simulink model "SPHERE_model4_Fuzzy"  (R2020a)
settings: Solver=ode4  StartTime=0.0  StopTime=30  FixedStep=0.01428571  RelTol=1e-3
values from neighbouring files (symbols this model uses):
  Final_val = 18    [Initial_script.m]    (also in Initial_script_test.m = -28; Initial_script_test2.m = -28)
  K = 25.937    [Initial_script.m]    (also in Initial_script_test.m; Initial_script_test2.m)
  L = -[ M2*l*(-2*l + R) - 2*J2, 0, -2*M2*l*g ]    [Initial_script.m]    (also in Initial_script_test.m; Initial_script_test2.m)
  M = [ J1 + 2*J2 + M1*R^2 + M2*(2*l^2 - 3*R*l + R^2), -Tv, 2*l*g*M2 ]    [Initial_script.m]    (also in Initial_script_test.m; Initial_script_test2.m)
  Smax = 502    [Initial_script.m]    (also in Initial_script_test.m; Initial_script_test2.m)
  Smin = -480    [Initial_script.m]    (also in Initial_script_test.m; Initial_script_test2.m)
  Step_time = 3.18    [Initial_script.m]    (also in Initial_script_test.m = 4.45; Initial_script_test2.m = 4.5)
  Top = 0.015    [Initial_script.m]    (also in Initial_script_test.m; Initial_script_test2.m)
undefined symbols (not defined in the file or in its folder): sigbuilder_block
libraries: fuzblock x1
settings Model: Creator=Adrian  LastModifiedBy=Adrian
settings OptimizationCC: DefaultParameterBehavior=Inlined  EnhancedBackFolding=on  PassReuseOutputArgsAs=Individual arguments  ZeroExternalMemoryAtStartup=off  ZeroInternalMemoryAtStartup=off  OptimizeBlockOrder=speed  DifferentSizesBufferReuse=on  OptimizationCustomize=off  EfficientTunableParamExpr=on
settings DebuggingCC: ParameterTunabilityLossMsg=error
settings SFSimCC: MATLABDynamicMemAlloc=off
settings RTWCC: SystemTargetFile=ert.tlc  TemplateMakefile=ert_default_tmf
settings CodeAppCC: ForceParamTrailComments=on  IgnoreCustomStorageClasses=off  OperatorAnnotations=on  SimulinkDataObjDesc=on  SFDataObjDesc=on  InsertBlockDesc=on
settings ERTTargetCC: TargetLangStandard=C99 (ISO)  GenerateSampleERTMain=on  InlinedParameterPlacement=NonHierarchical  ERTCustomFileTemplate=example_file_process.tlc

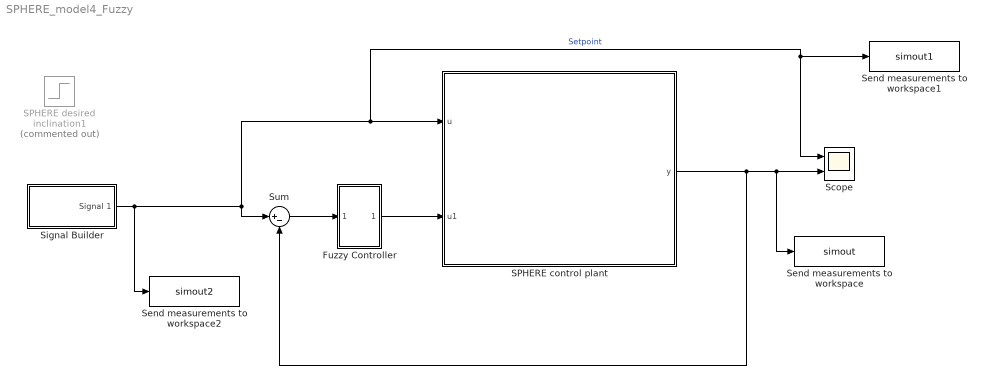
== system SPHERE_model4_Fuzzy ==
  Fuzzy Controller : Subsystem
  SPHERE control plant : Subsystem
      mask Display: image('C:\Users\Adrian\Documents\Praca Magisterska\Robot kulisty by Adrian\Praca Magisterska\LaTex\Pictures\Old\sphere_full.PNG'); % Use "Edit Image" on toolstrip to change.
  SPHERE desired inclination1 : Step  Commented=on  Time=Step_time  After=Final_val  SampleTime=0
  Scope : Scope  NumInputPorts=2
  Send measurements to workspace : ToWorkspace  VariableName=simout  SaveFormat=Timeseries  SampleTime=-1
  Send measurements to workspace1 : ToWorkspace  VariableName=simout1  SaveFormat=Timeseries  SampleTime=-1
  Send measurements to workspace2 : ToWorkspace  VariableName=simout2  SaveFormat=Timeseries  SampleTime=-1
  Signal Builder : Subsystem  Tag=STV Subsys  LoadFcn=sigbuilder_block('load');  StartFcn=sigbuilder_block('start');  StopFcn=sigbuilder_block('stop');  ClipboardFcn=sigbuilder_block('clipboard');  mask(Sigbuilder block){tuvar=[0:10]}
      mask help: Simulink:masks:SigbuilderBlock_MD
      mask init:
      | if ~strcmp(get_param(bdroot(gcbh),'SimulationStatus'),'stopped') tuvar = sigbuilder_block('maskInit'); end
      settings: CopyFcn=sigbuilder_block('copy');  DeleteFcn=sigbuilder_block('delete');  ModelCloseFcn=sigbuilder_block('modelClose');  PreSaveFcn=sigbuilder_block('preSave');  PauseFcn=sigbuilder_block('pause');  ContinueFcn=sigbuilder_block('continue');  NameChangeFcn=sigbuilder_block('namechange');  OpenFcn=sigbuilder_block('open',[90.75 122.25 550.5 399.75 ]);  CloseFcn=sigbuilder_block('close');
      mask Display: plot(0, 0, 100, 100,[2, 2, 32, 32, 2], [68, 8, 8, 68, 68],[32, 2], [38, 38], [32, 19, 2],[53, 60, 44], [32, 17, 17, 2],[16, 16, 31, 31]);txt = getActiveGroup(gcbh);text(2, 100, txt,'verticalAlignment', 'top');
  Sum : Sum  Inputs=|+-
  wires:
  SPHERE control plant/1(y) -> Sum/2, Send measurements to workspace/1, Scope/2
  Signal Builder/1(Signal 1) -> Send measurements to workspace2/1, Sum/1, Send measurements to workspace1/1, Scope/1, SPHERE control plant/1(u)  "Setpoint"
  Sum/1 -> Fuzzy Controller/1(In1)
  Fuzzy Controller/1(Out1) -> SPHERE control plant/2(u1)

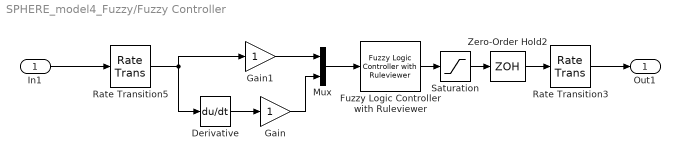
== system SPHERE_model4_Fuzzy/Fuzzy Controller ==
  In1 : Inport
  Derivative : Derivative
  Fuzzy Logic Controller with Ruleviewer : fuzblock/Fuzzy Logic  Controller  with Ruleviewer  fismatrix=FUZZY_controller5  Ts=0.07142855
  Gain : Gain
  Gain1 : Gain
  Mux : Mux  Inputs=2
  Rate Transition3 : RateTransition
  Rate Transition5 : RateTransition
  Saturation : Saturate  UpperLimit=60  LowerLimit=-60
  Zero-Order Hold2 : ZeroOrderHold  SampleTime=-1
  Out1 : Outport
  wires:
  In1/1 -> Rate Transition5/1
  Rate Transition3/1 -> Out1/1
  Gain/1 -> Mux/2
  Zero-Order Hold2/1 -> Rate Transition3/1
  Gain1/1 -> Mux/1
  Rate Transition5/1 -> Derivative/1, Gain1/1
  Saturation/1 -> Zero-Order Hold2/1
  Derivative/1 -> Gain/1
  Fuzzy Logic Controller with Ruleviewer/1 -> Saturation/1
  Mux/1 -> Fuzzy Logic Controller with Ruleviewer/1

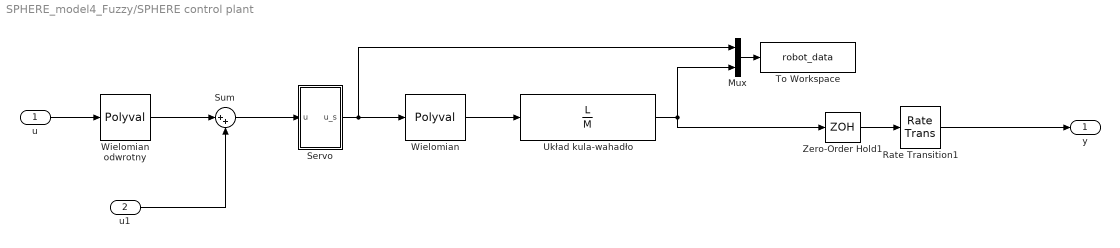
== system SPHERE_model4_Fuzzy/SPHERE control plant ==
  u : Inport
  u1 : Inport  Port=2
  Mux : Mux  Inputs=2
  Rate Transition1 : RateTransition
  Servo : Subsystem
  Sum : Sum  Inputs=|++
  To Workspace : ToWorkspace  VariableName=robot_data  SaveFormat=Structure With Time  SampleTime=-1
  Układ kula-wahadło : TransferFcn  Numerator=L  Denominator=M
  Wielomian : Polyval  Coefs=[-0.000067 -0.000287 0.871698 0]
  Wielomian odwrotny : Polyval  Coefs=[0.000325 0.001274 1.044515 0]
  Zero-Order Hold1 : ZeroOrderHold  SampleTime=-1
  y : Outport
  wires:
  Układ kula-wahadło/1 -> Mux/2, Zero-Order Hold1/1
  Servo/1(u_s) -> Wielomian/1, Mux/1
  Mux/1 -> To Workspace/1
  Zero-Order Hold1/1 -> Rate Transition1/1
  Rate Transition1/1 -> y/1
  Wielomian/1 -> Układ kula-wahadło/1
  Sum/1 -> Servo/1(u)
  Wielomian odwrotny/1 -> Sum/1
  u1/1 -> Sum/2
  u/1 -> Wielomian odwrotny/1

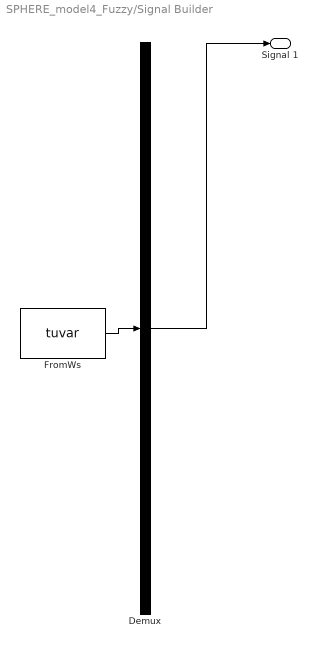
== system SPHERE_model4_Fuzzy/Signal Builder ==
  Demux : Demux  Tag=STV Demux  Outputs=1
      settings: DisplayOption=none
  FromWs : FromWorkspace  Tag=STV FromWs  VariableName=tuvar
      SigBuilderData=|
      | common.afterFinalStr = 'Extrapolate'
      | common.sampleTime = 0
      | dataSet.timeRange = [0 30]
      | dataSet.name = 'Group 1'
      | sbobj.Groups.Name = 'Group 1'
      | sbobj.Groups.Signals.Name = 'Signal 1'
      | sbobj.Groups.Signals.XData = [0 1 1 15 15 30]
      | sbobj.Groups.Signals.YData = [0 0.005 15 15 -15 -15]
      | sbobj.Groups.TimeRange = [0 30]
  Signal 1 : Outport  Tag=STV Outport
  wires:
  Demux/1 -> Signal 1/1
  FromWs/1 -> Demux/1

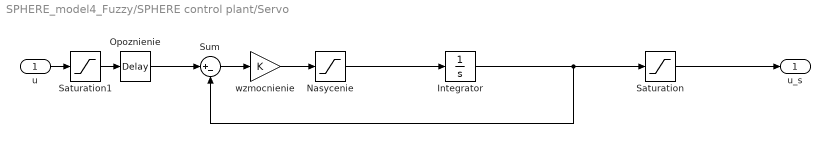
== system SPHERE_model4_Fuzzy/SPHERE control plant/Servo ==
  u : Inport
  Integrator : Integrator
  Nasycenie : Saturate  UpperLimit=Smax  LowerLimit=Smin
  Opoznienie : TransportDelay  DelayTime=Top
  Saturation : Saturate  UpperLimit=60  LowerLimit=-60
  Saturation1 : Saturate  UpperLimit=60  LowerLimit=-60
  Sum : Sum  Inputs=|+-
  wzmocnienie : Gain  Gain=K
  u_s : Outport
  wires:
  Sum/1 -> wzmocnienie/1
  Integrator/1 -> Saturation/1, Sum/2
  wzmocnienie/1 -> Nasycenie/1
  Opoznienie/1 -> Sum/1
  Nasycenie/1 -> Integrator/1
  u/1 -> Saturation1/1
  Saturation/1 -> u_s/1
  Saturation1/1 -> Opoznienie/1
